simulink model "example03"  (R2022a)
settings: Solver=VariableStepAuto  StartTime=0.0  StopTime=10.0  RelTol=1e-3
settings Model: Creator=cunis  LastModifiedBy=cunis

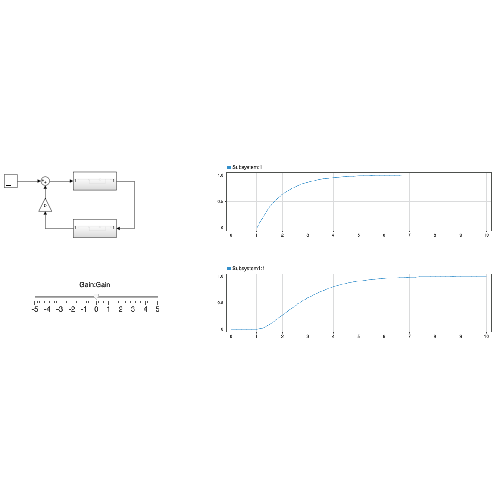
[thumbnail: Simulink's stored preview of the top-level diagram]
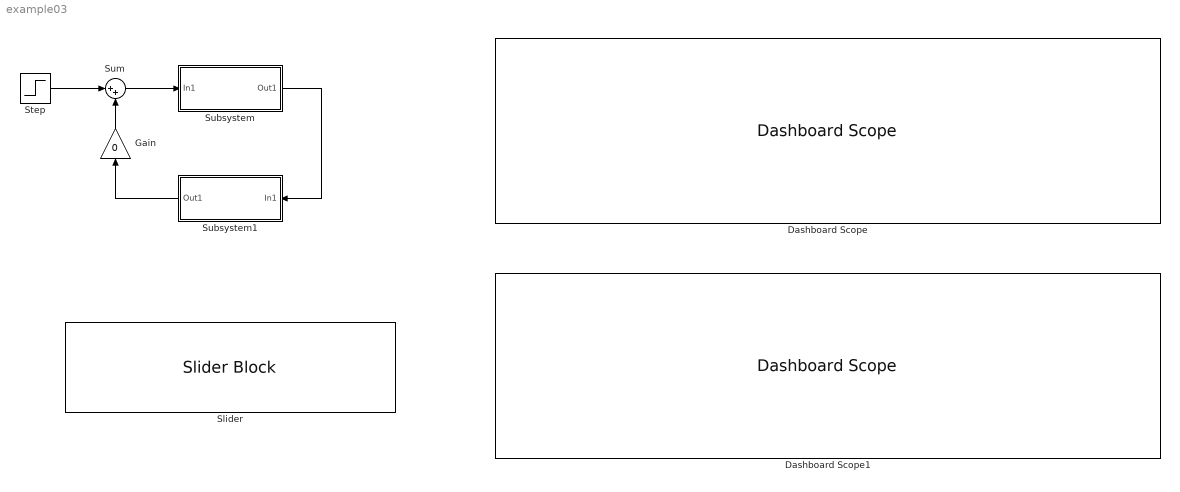
== system example03 ==
  Dashboard Scope : DashboardScope
  Dashboard Scope1 : DashboardScope
  Gain : Gain  Gain=0
  Slider : SliderBlock  ScaleMin=-5  ScaleMax=5
  Step : Step  SampleTime=0
  Subsystem : Subsystem
  Subsystem1 : Subsystem
  Sum : Sum  Inputs=|++
  wires:
  Step/1 -> Sum/1
  Sum/1 -> Subsystem/1(In1)
  Subsystem/1(Out1) -> Subsystem1/1(In1)
  Gain/1 -> Sum/2
  Subsystem1/1(Out1) -> Gain/1

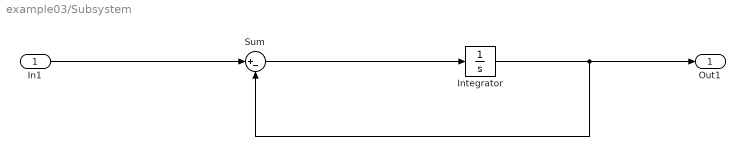
== system example03/Subsystem ==
  In1 : Inport
  Integrator : Integrator
  Sum : Sum  Inputs=|+-
  Out1 : Outport
  wires:
  In1/1 -> Sum/1
  Sum/1 -> Integrator/1
  Integrator/1 -> Sum/2, Out1/1

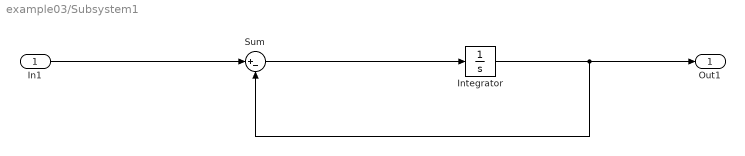
== system example03/Subsystem1 ==
  In1 : Inport
  Integrator : Integrator
  Sum : Sum  Inputs=|+-
  Out1 : Outport
  wires:
  Integrator/1 -> Out1/1, Sum/2
  Sum/1 -> Integrator/1
  In1/1 -> Sum/1
